simulink model "FV_tolga_catalbas_odev1"  (R2018a)
settings: Solver=VariableStepAuto  StartTime=0.0  StopTime=4  RelTol=1e-3
values from neighbouring files (symbols this model uses):
  n = n+1    (= 1)    [LVQ_kodu.m]    (also in MLNN1_kodu.m; MLNN2_kodu.m; pnn_kodu.m)
undefined symbols (not defined in the file or in its folder): Eg0, Isc, K, ki, Ns, q, Rs, Rsh, Tn, Voc
libraries: simulink x3
settings Model: Creator=Tolga  LastModifiedBy=Tolga

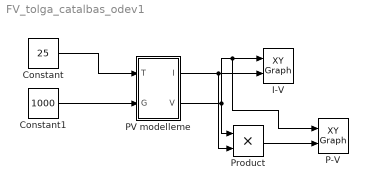
== system FV_tolga_catalbas_odev1 ==
  Constant : Constant  Value=25
  Constant1 : Constant  Value=1000
  I-V : simulink/Sinks/XY Graph  xmin=0  xmax=35  ymin=0  ymax=10  st=-1
  P-V : simulink/Sinks/XY Graph  xmin=0  xmax=35  ymin=0  ymax=210  st=-1
  PV modelleme : Subsystem  InitFcn=|
      | ki=.0032,
      | q=1.6e-19,
      | K=1.38e-23,
      | n=1.3,
      | Eg0=1.1,
      | Rs=.221,
      | Rsh=415.405,
      | Tn=298,
      | Voc=32.9,
      | Isc=8.21,
      | Ns=54,
  Product : Product
  wires:
  Constant1/1 -> PV modelleme/2(G)
  Constant/1 -> PV modelleme/1(T)
  PV modelleme/1(I) -> Product/2, I-V/2
  PV modelleme/2(V) -> Product/1, P-V/1, I-V/1
  Product/1 -> P-V/2

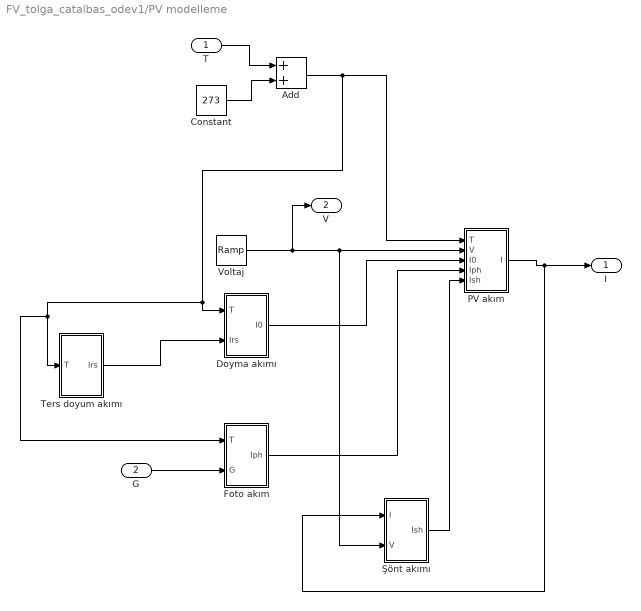
== system FV_tolga_catalbas_odev1/PV modelleme ==
  T : Inport
  G : Inport  Port=2
  Add : Sum
  Constant : Constant  Value=273
  Doyma akımı : Subsystem
  Foto akım : Subsystem
  PV akım : Subsystem
  Ters doyum akımı : Subsystem
  Voltaj : simulink/Sources/Ramp  slope=10  start=0  InitialOutput=0
  Şönt akımı : Subsystem
  I : Outport
  V : Outport  Port=2
  wires:
  Şönt akımı/1(Ish) -> PV akım/5(Ish)
  Add/1 -> Foto akım/1(T), Ters doyum akımı/1(T), Doyma akımı/1(T), PV akım/1(T)
  Foto akım/1(Iph) -> PV akım/4(Iph)
  Doyma akımı/1(I0) -> PV akım/3(I0)
  Voltaj/1 -> V/1, Şönt akımı/2("V "), PV akım/2(V)
  Constant/1 -> Add/2
  Ters doyum akımı/1(Irs) -> Doyma akımı/2(Irs)
  PV akım/1(I) -> I/1, Şönt akımı/1("I ")
  G/1 -> Foto akım/2(G)
  T/1 -> Add/1

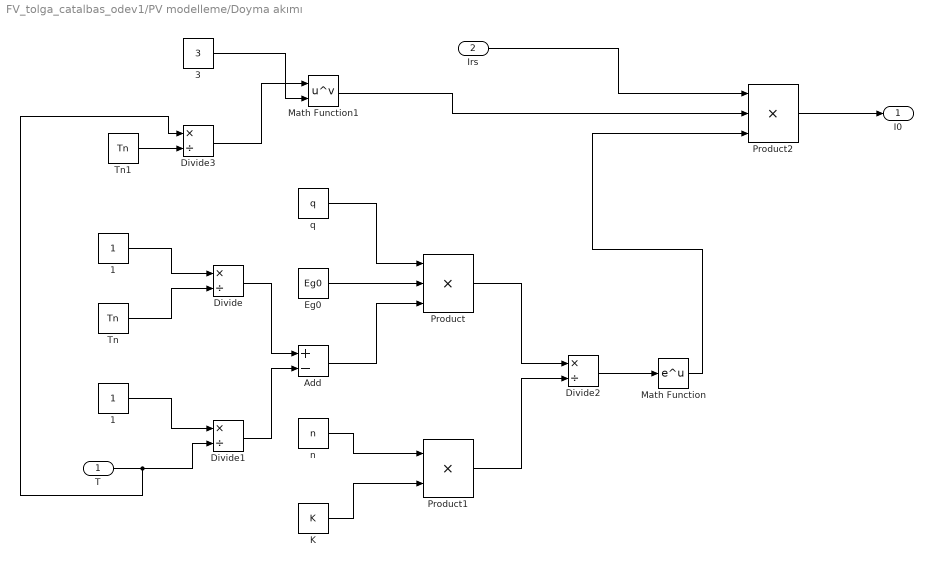
== system FV_tolga_catalbas_odev1/PV modelleme/Doyma akımı ==
  T : Inport
  Irs : Inport  Port=2
  1 : Constant
  "1 " : Constant
  3 : Constant  Value=3
  Add : Sum  Inputs=+-
  Divide{,1..3} (4 alike) : Product  Inputs=*/
  Eg0 : Constant  Value=Eg0
  K : Constant  Value=K
  Math Function : Math  SaturateOnIntegerOverflow=on
  Math Function1 : Math  Operator=pow  SaturateOnIntegerOverflow=on
  Product : Product  Inputs=3
  Product1 : Product
  Product2 : Product  Inputs=3
  Tn : Constant  Value=Tn
  Tn1 : Constant  Value=Tn
  n : Constant  Value=n
  q : Constant  Value=q
  I0 : Outport
  wires:
  Divide/1 -> Add/1
  Irs/1 -> Product2/1
  Tn1/1 -> Divide3/2
  "1 "/1 -> Divide/1
  n/1 -> Product1/1
  3/1 -> Math Function1/2
  Tn/1 -> Divide/2
  Math Function/1 -> Product2/3
  Product2/1 -> I0/1
  Product/1 -> Divide2/1
  1/1 -> Divide1/1
  Math Function1/1 -> Product2/2
  K/1 -> Product1/2
  q/1 -> Product/1
  T/1 -> Divide1/2, Divide3/1
  Product1/1 -> Divide2/2
  Divide1/1 -> Add/2
  Divide3/1 -> Math Function1/1
  Add/1 -> Product/3
  Divide2/1 -> Math Function/1
  Eg0/1 -> Product/2

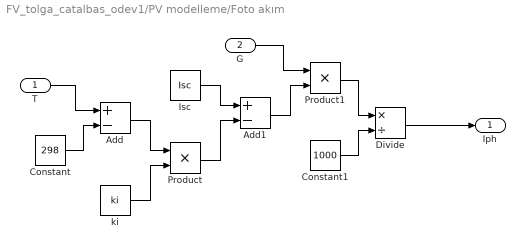
== system FV_tolga_catalbas_odev1/PV modelleme/Foto akım ==
  T : Inport
  G : Inport  Port=2
  Add : Sum  Inputs=+-
  Add1 : Sum  Inputs=+-
  Constant : Constant  Value=298
  Constant1 : Constant  Value=1000
  Divide : Product  Inputs=*/
  Isc : Constant  Value=Isc
  Product : Product
  Product1 : Product
  ki : Constant  Value=ki
  Iph : Outport
  wires:
  Constant/1 -> Add/2
  Isc/1 -> Add1/1
  Add/1 -> Product/1
  Constant1/1 -> Divide/2
  ki/1 -> Product/2
  Product1/1 -> Divide/1
  T/1 -> Add/1
  G/1 -> Product1/1
  Add1/1 -> Product1/2
  Divide/1 -> Iph/1
  Product/1 -> Add1/2

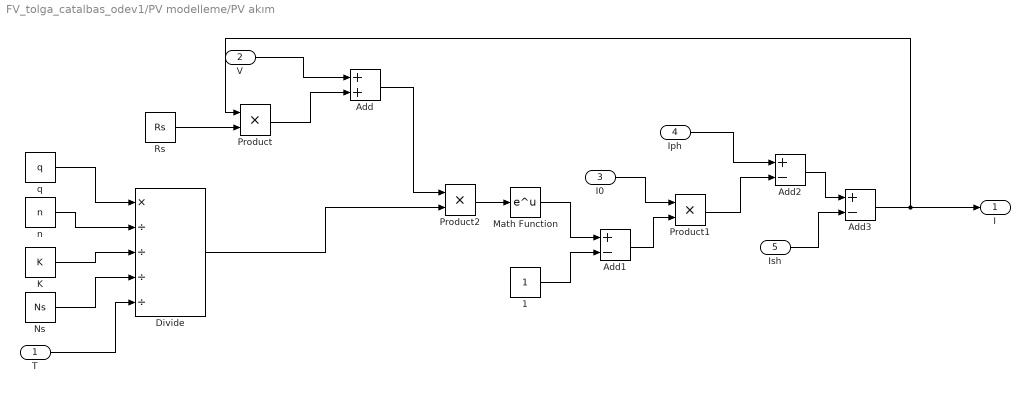
== system FV_tolga_catalbas_odev1/PV modelleme/PV akım ==
  T : Inport
  V : Inport  Port=2
  I0 : Inport  Port=3
  Iph : Inport  Port=4
  Ish : Inport  Port=5
  1 : Constant
  Add : Sum
  Add1 : Sum  Inputs=+-
  Add2 : Sum  Inputs=+-
  Add3 : Sum  Inputs=+-
  Divide : Product  Inputs=*////
  K : Constant  Value=K
  Math Function : Math  SaturateOnIntegerOverflow=on
  Ns : Constant  Value=Ns
  Product : Product
  Product1 : Product
  Product2 : Product
  Rs : Constant  Value=Rs
  n : Constant  Value=n
  q : Constant  Value=q
  I : Outport
  wires:
  Product2/1 -> Math Function/1
  I0/1 -> Product1/1
  V/1 -> Add/1
  Add3/1 -> I/1, Product/1
  Add/1 -> Product2/1
  Ish/1 -> Add3/2
  Iph/1 -> Add2/1
  Ns/1 -> Divide/4
  Divide/1 -> Product2/2
  Add2/1 -> Add3/1
  n/1 -> Divide/2
  T/1 -> Divide/5
  Product/1 -> Add/2
  Add1/1 -> Product1/2
  Rs/1 -> Product/2
  1/1 -> Add1/2
  Math Function/1 -> Add1/1
  K/1 -> Divide/3
  Product1/1 -> Add2/2
  q/1 -> Divide/1

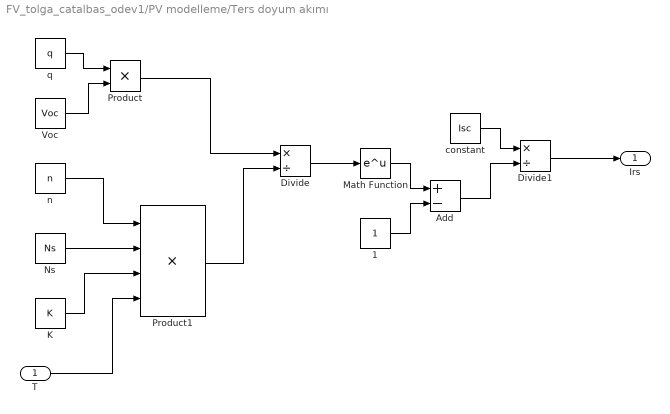
== system FV_tolga_catalbas_odev1/PV modelleme/Ters doyum akımı ==
  T : Inport
  1 : Constant
  Add : Sum  Inputs=+-
  Divide : Product  Inputs=*/
  Divide1 : Product  Inputs=*/
  K : Constant  Value=K
  Math Function : Math  SaturateOnIntegerOverflow=on
  Ns : Constant  Value=Ns
  Product : Product
  Product1 : Product  Inputs=4
  Voc : Constant  Value=Voc
  constant : Constant  Value=Isc
  n : Constant  Value=n
  q : Constant  Value=q
  Irs : Outport
  wires:
  T/1 -> Product1/4
  Product/1 -> Divide/1
  Divide/1 -> Math Function/1
  1/1 -> Add/2
  Divide1/1 -> Irs/1
  q/1 -> Product/1
  Ns/1 -> Product1/2
  Math Function/1 -> Add/1
  Add/1 -> Divide1/2
  Voc/1 -> Product/2
  K/1 -> Product1/3
  n/1 -> Product1/1
  Product1/1 -> Divide/2
  constant/1 -> Divide1/1

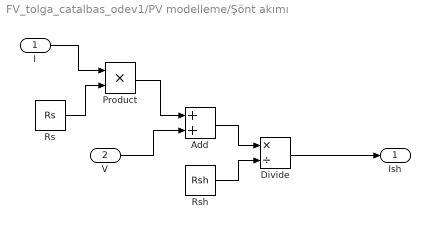
== system FV_tolga_catalbas_odev1/PV modelleme/Şönt akımı ==
  "I " : Inport
  "V " : Inport  Port=2
  Add : Sum
  Divide : Product  Inputs=*/
  Product : Product
  Rs : Constant  Value=Rs
  Rsh : Constant  Value=Rsh
  Ish : Outport
  wires:
  "I "/1 -> Product/1
  Add/1 -> Divide/1
  "V "/1 -> Add/2
  Rsh/1 -> Divide/2
  Rs/1 -> Product/2
  Product/1 -> Add/1
  Divide/1 -> Ish/1
